simulink model "STEVE_Simulation"  (R2024b)
settings: Solver=ode4  StartTime=0.0  StopTime=60*6  FixedStep=0.05  RelTol=1e-3  EnableMultiTasking=on
values from neighbouring files (symbols this model uses):
  F = scatteredInterpolant(obj.MachData, obj.AlphaData, obj.CLData, obj.InterpMethod, 'none')    [LookupInitializer.m]
  rocket_length = max(STeVe_Contour.X) - min(STeVe_Contour.X)    [initialize_parameters.m]
  timeStep = 0.005    [initialize_parameters.m]
undefined symbols (not defined in the file or in its folder): Actuators, AeroData, Earth, Light, MIL, PrelookupData, Ref_Area, WGS84
libraries: aerolibwind2 x3, aerolibtransform2 x3, aerolibasang x3, simulink x1, aerolibatmos2 x1, simulink_extras x1, slpidlib x1, aerolibconvert2 x1, aerolibactuator x1
settings Model: ExtModeTrigDuration=2  Creator=jonno  LastModifiedBy=jonno
settings SolverCC: AutoInsertRateTranBlk=on
settings RTWCC: BuildConfiguration=Faster Runs

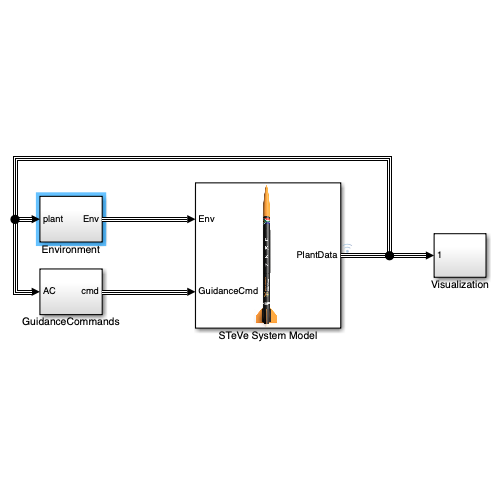
[thumbnail: Simulink's stored preview of the top-level diagram]
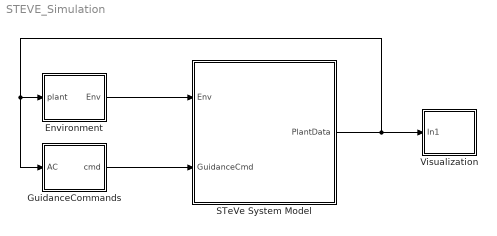
== system STEVE_Simulation ==
  Environment : Subsystem
  GuidanceCommands : Subsystem
  STeVe System Model : Subsystem
      mask Display: image('steve.png', [65 - (50 * (187 / 1041)), 0, 140 * (187 / 1041), 140])
  Visualization : Subsystem
  wires:
  GuidanceCommands/1(cmd) -> STeVe System Model/2(GuidanceCmd)
  Environment/1(Env) -> STeVe System Model/1(Env)
  STeVe System Model/1(PlantData) -> GuidanceCommands/1(AC), Environment/1(plant), Visualization/1(In1)

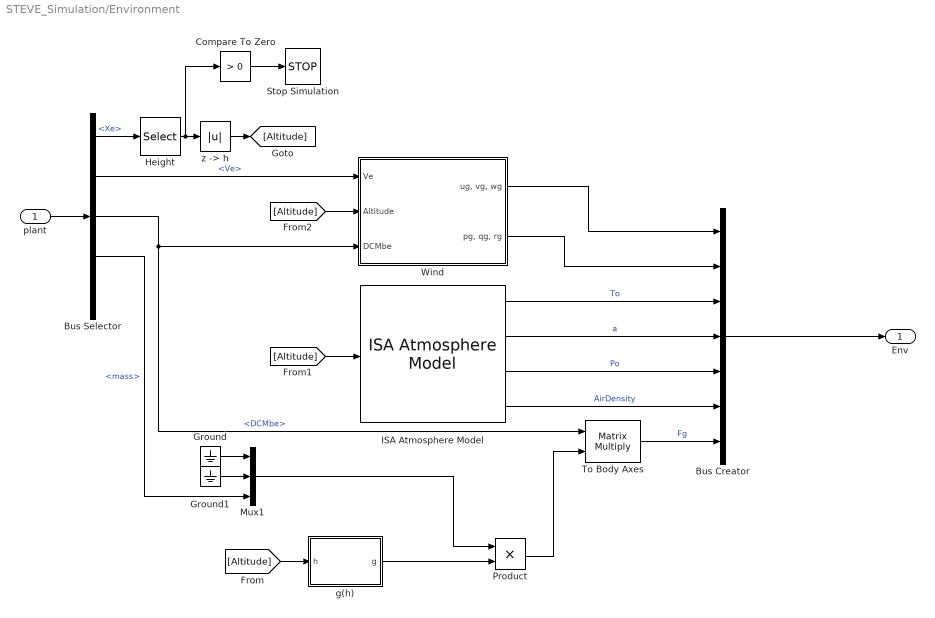
== system STEVE_Simulation/Environment ==
  plant : Inport
  Bus Creator : BusCreator  Inputs=7
  Bus Selector : BusSelector  OutputSignals=Xe,Ve,DCMbe,mass,lat
  Compare To Zero : simulink/Logic and Bit Operations/Compare To Zero  relop=>  OutDataTypeStr=boolean
  Ground : Ground
  Ground1 : Ground
  Height : Selector  IndexMode=Zero-based  InputPortWidth=3  IndexOptions=Index vector (dialog)  Indices=2  OutputSizes=1
  ISA Atmosphere Model : aerolibatmos2/ISA Atmosphere Model  useExtended=on  action=None  custom=off  viscosityOut=off  g=9.80665  gamma=1.4  R=287.0531  L=0.0065  h_trop=11000  h_strat=20000  rho0=1.225  P0=101325  T0=288.15  h0=0  S=110.4  Tref=273.15  muref=1.716e-5
  Mux1 : Mux  Inputs=3
  Product : Product
  Stop Simulation : Stop
  To Body Axes : Product  Multiplication=Matrix(*)
  Wind : Subsystem
  g(h) : MATLAB Function  TreatAsAtomicUnit=on
  "z -> h" : Abs  SaturateOnIntegerOverflow=off
  Env : Outport
  wires:
  plant/1 -> Bus Selector/1
  Bus Creator/1 -> Env/1
  Compare To Zero/1 -> Stop Simulation/1
  Bus Selector/1 -> Height/1  "<Xe>"
  Height/1 -> Compare To Zero/1, "z -> h"/1
  "z -> h"/1 -> [Altitude]
  Bus Selector/4 -> Mux1/3  "<mass>"
  Ground/1 -> Mux1/1
  Ground1/1 -> Mux1/2
  Bus Selector/3 -> Wind/3(DCMbe), To Body Axes/1  "<DCMbe>"
  [Altitude] -> ISA Atmosphere Model/1
  To Body Axes/1 -> Bus Creator/7  "Fg"
  ISA Atmosphere Model/4 -> Bus Creator/6  "AirDensity"
  ISA Atmosphere Model/3 -> Bus Creator/5  "Po"
  ISA Atmosphere Model/2 -> Bus Creator/4  "a"
  ISA Atmosphere Model/1 -> Bus Creator/3  "To"
  Bus Selector/2 -> Wind/1(Ve)  "<Ve>"
  [Altitude] -> Wind/2(Altitude)
  Wind/2("pg, qg, rg") -> Bus Creator/2
  Wind/1("ug, vg, wg") -> Bus Creator/1
  Mux1/1 -> Product/1
  Product/1 -> To Body Axes/2
  [Altitude] -> g(h)/1(h)
  g(h)/1(g) -> Product/2

== system STEVE_Simulation/GuidanceCommands ==
  AC : Inport
  Bus Creator : BusCreator  Inputs=2
  Degrees to Radians : simulink_extras/Transformations/Degrees to Radians
  Rate Limiter : RateLimiter  SampleTimeMode=inherited
  Terminator : Terminator
  ThetaCmd : Step  Before=90  After=90  SampleTime=0
  ThrottleCmd %1 : Step  Time=Actuators.Engine.BurnTime  Before=1  After=0  SampleTime=0
  cmd : Outport
  wires:
  AC/1 -> Terminator/1
  ThrottleCmd %1/1 -> Rate Limiter/1
  Bus Creator/1 -> cmd/1
  ThetaCmd/1 -> Degrees to Radians/1  "ThetaCmd"
  Degrees to Radians/1 -> Bus Creator/2  "ThetaCmd"
  Rate Limiter/1 -> Bus Creator/1  "ThrottleCmd"

== system STEVE_Simulation/STeVe System Model ==
  Env : Inport
  GuidanceCmd : Inport  Port=2
  Avionics : Subsystem
  Env1 : InportShadow
  Flight Sensors : Subsystem
  Vehicle : Subsystem
  PlantData : Outport
  wires:
  Env/1 -> Vehicle/1(Env)
  Vehicle/1(PlantData) -> Flight Sensors/2(Plant), Avionics/2(PlantData), PlantData/1  "Plant"
  Avionics/1(ActCmd) -> Vehicle/2(ActCmd)
  GuidanceCmd/1 -> Avionics/1(GuidanceCommandBus)
  Env1/1 -> Flight Sensors/1(Env)
  Flight Sensors/1(Sensors) -> Avionics/3(Sensors)

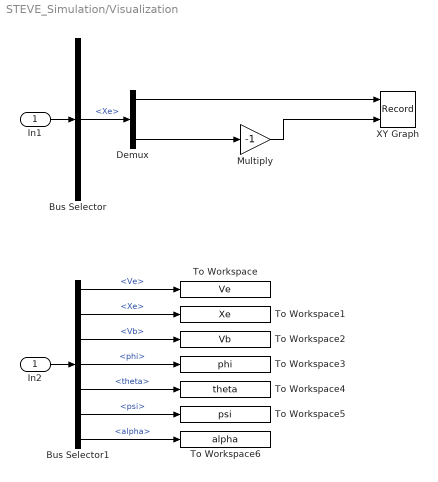
== system STEVE_Simulation/Visualization ==
  In1 : Inport
  Bus Selector : BusSelector  OutputSignals=Xe
  Bus Selector1 : BusSelector  OutputSignals=Ve,Xe,Vb,body angles.phi,body angles.theta,body angles.psi,alpha
  Demux : Demux  Outputs=3
  In2 : InportShadow
  Multiply : Gain  Gain=-1
  To Workspace : ToWorkspace  VariableName=Ve  SaveFormat=Timeseries  SampleTime=-1
  To Workspace1 : ToWorkspace  VariableName=Xe  SaveFormat=Timeseries  SampleTime=-1
  To Workspace2 : ToWorkspace  VariableName=Vb  SaveFormat=Timeseries  SampleTime=-1
  To Workspace3 : ToWorkspace  VariableName=phi  SaveFormat=Timeseries  SampleTime=-1
  To Workspace4 : ToWorkspace  VariableName=theta  SaveFormat=Timeseries  SampleTime=-1
  To Workspace5 : ToWorkspace  VariableName=psi  SaveFormat=Timeseries  SampleTime=-1
  To Workspace6 : ToWorkspace  VariableName=alpha  SaveFormat=Timeseries  SampleTime=-1
  XY Graph : Record  FileSettingsInternal="{\"entries\":[{\"content\":{\"excelSettings\":{\"content\":{},\"type\":\"Streamout.ExcelSettings\"}},\"type\":\"Streamout.FileSettingStorage\",\"uuid\":\"\"}],\"packageUris\":[\"http:\\/\\/schema.mathworks.com\\/mf0\\/streamout_blocks\\/R2020a\"],\"version\":\"1.0\"}"  Layout=[1 1]  SignalsInternal="{\"entries\":[{\"content\":{\"signals\":[{\"content\":{\"blockPath\":[],\"dimensions\":[1],\"domain\":\"\",\"lineColor\":\"#a2142f\",\"plots\":[ 1 ],\"port\":1,\"sid\":[\"\"],\"signalID\":1,\"signalName\":\"Demux:1\"},\"type\":\"RecordBlkView.Signal\",\"uuid\":\"\"},{\"content\":{\"blockPath\":[],\"dimensions\":[1],\"domain\":\"\",\"lineColor\":\"#139fff\",\"plots\":[ 1 ],\"port\":2,\"sid\":[\"\"],\"signalID\":2,\"signalName\":\"Multiply\"},\"type\":\"RecordBlkView.Signal\",\"uuid\":\"\"}]},\"type\":\"RecordBlkView.InputSignals\",\"uuid\":\"\"}],\"packageUris\":[\"http:\\/\\/schema.mathworks.com\\/mf0\\/streamout_blocks\\/R2020a\"],\"version\":\"1.0\"}"  VisualizationBindings="{\"xyplotplugin\":{\"info\":[{\"series\":[{\"bindingParametersList\":[{\"parameter\":\"X-Axis\",\"signalID\":1,\"signalName\":\"Demux:1\"},{\"parameter\":\"Y-Axis\",\"signalID\":2,\"signalName\":\"Multiply\"}],\"seriesID\":0}],\"subplotID\":1}]}}"  CompatibilityTag=XY
  wires:
  In1/1 -> Bus Selector/1
  Bus Selector/1 -> Demux/1  "<Xe>"
  Multiply/1 -> XY Graph/2
  Demux/3 -> Multiply/1
  Demux/1 -> XY Graph/1
  In2/1 -> Bus Selector1/1
  Bus Selector1/1 -> To Workspace/1  "<Ve>"
  Bus Selector1/2 -> To Workspace1/1  "<Xe>"
  Bus Selector1/3 -> To Workspace2/1  "<Vb>"
  Bus Selector1/4 -> To Workspace3/1  "<phi>"
  Bus Selector1/5 -> To Workspace4/1  "<theta>"
  Bus Selector1/6 -> To Workspace5/1  "<psi>"
  Bus Selector1/7 -> To Workspace6/1  "<alpha>"

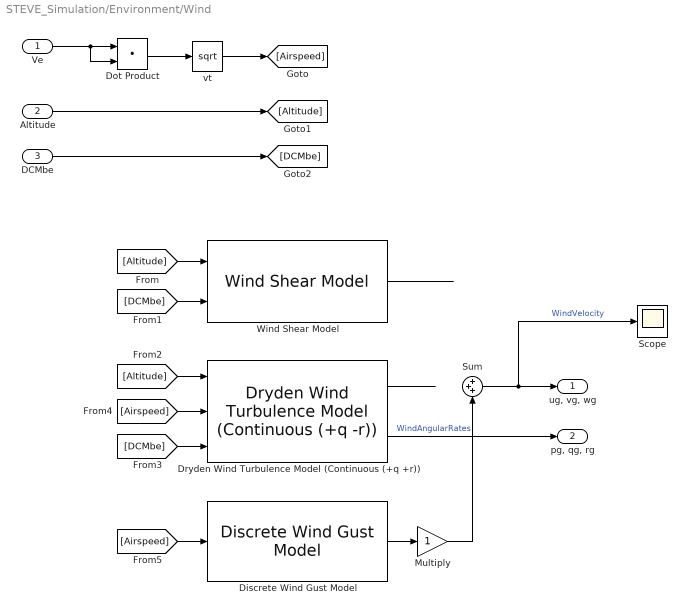
== system STEVE_Simulation/Environment/Wind ==
  Ve : Inport
  Altitude : Inport  Port=2
  DCMbe : Inport  Port=3
  Discrete Wind Gust Model : aerolibwind2/Discrete Wind Gust Model  units=Metric (MKS)  Gx=on  Gy=on  Gz=on  t_0=2  d_m=[120 100 80]  v_m=[3.5 4.0 3.0]
  Dot Product : DotProduct  OutDataTypeStr=Inherit: Inherit via internal rule
  Dryden Wind Turbulence Model (Continuous (+q +r)) : aerolibwind2/Dryden Wind Turbulence Model  (Continuous (+q -r))  units=Metric (MKS)  spec=MIL-F-8785C  model=Continuous Dryden (+q +r)  W20=15  Wdeg=0  TurbProb=10^-2 - Light  L_high=533.4  Wingspan=10  ts=0.1  Seed=[23341 23342 23343 23344]  T_on=off
      settings: LibrarySourceBlock=|
      | aerolibwind2/Dryden Wind Turbulence Model
      | (Continuous (+q +r))
  Multiply : Gain
  Scope : Scope
  Sum : Sum  Inputs=+++
  Wind Shear Model : aerolibwind2/Wind Shear Model  units=Metric (MKS)  phase=Category C - Terminal Flight Phase  W_20=1  Wdeg=0
  vt : Sqrt
  "ug, vg, wg" : Outport
  "pg, qg, rg" : Outport  Port=2
  wires:
  Ve/1 -> Dot Product/2, Dot Product/1
  Dot Product/1 -> vt/1
  vt/1 -> [Airspeed]
  DCMbe/1 -> [DCMbe]
  [Altitude] -> Wind Shear Model/1
  [DCMbe] -> Wind Shear Model/2
  [Altitude] -> Dryden Wind Turbulence Model (Continuous (+q +r))/1
  [DCMbe] -> Dryden Wind Turbulence Model (Continuous (+q +r))/3
  [Airspeed] -> Dryden Wind Turbulence Model (Continuous (+q +r))/2
  [Airspeed] -> Discrete Wind Gust Model/1
  Discrete Wind Gust Model/1 -> Multiply/1
  Wind Shear Model/1 -> ?
  Sum/1 -> Scope/1, "ug, vg, wg"/1  "WindVelocity"
  Dryden Wind Turbulence Model (Continuous (+q +r))/2 -> "pg, qg, rg"/1  "WindAngularRates"
  Altitude/1 -> [Altitude]
  Dryden Wind Turbulence Model (Continuous (+q +r))/1 -> ?
  Multiply/1 -> Sum/3

== system STEVE_Simulation/STeVe System Model/Avionics ==
  GuidanceCommandBus : Inport
  PlantData : Inport  Port=2
  Sensors : Inport  Port=3
  Bus Selector : BusSelector  OutputSignals=body angles.theta,w
  ControlSystem : Subsystem
  Scope : Scope
  ActCmd : Outport
  wires:
  PlantData/1 -> Bus Selector/1
  GuidanceCommandBus/1 -> ControlSystem/2(Guidance)
  ControlSystem/1(cmd) -> ActCmd/1
  Sensors/1 -> ?
  Bus Selector/1 -> ControlSystem/1(AvionicsBus), Scope/1  "<theta>"

== system STEVE_Simulation/STeVe System Model/Flight Sensors ==
  Env : Inport
  Plant : Inport  Port=2
  Sensors : Outport
  wires:
  Plant/1 -> ?

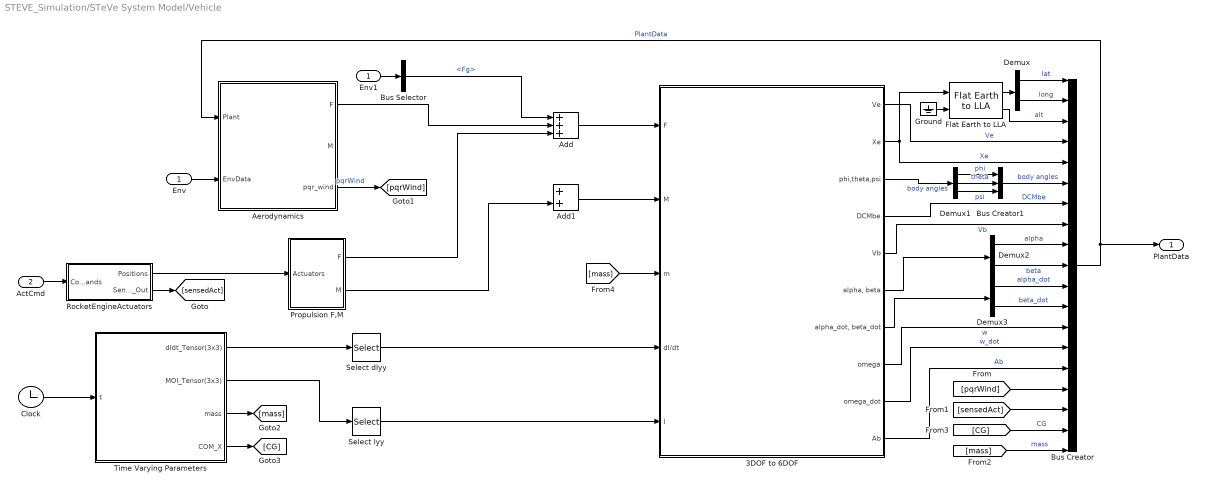
== system STEVE_Simulation/STeVe System Model/Vehicle ==
  Env : Inport
  ActCmd : Inport  Port=2
  3DOF to 6DOF : Subsystem
  Add : Sum  Inputs=+++
  Add1 : Sum
  Aerodynamics : Subsystem
  Bus Creator : BusCreator  Inputs=19
  Bus Creator1 : BusCreator  Inputs=3
  Bus Selector : BusSelector  OutputSignals=Fg
  Clock : Clock
  Demux : Demux  Outputs=2
  Demux1 : Demux  Outputs=3
  Demux2 : Demux  Outputs=2
  Demux3 : Demux  Outputs=2
  Env1 : InportShadow
  Flat Earth to LLA : aerolibtransform2/Flat Earth to LLA  units=Metric (MKS)  ptype=Earth (WGS84)  F=1/298.257223563  R=6378137  refPosPort=off  LL0=[0 10]  psi=0
  Ground : Ground
  Propulsion F,M : Subsystem
  RocketEngineActuators : Subsystem
  Select Iyy : Selector  NumberOfDimensions=2  InputPortWidth=3  IndexOptions=Index vector (dialog),Index vector (dialog)  Indices=[1],[1]  OutputSizes=1,1
  Select dIyy : Selector  NumberOfDimensions=2  InputPortWidth=3  IndexOptions=Index vector (dialog),Index vector (dialog)  Indices=[1],[1]  OutputSizes=1,1
  Time Varying Parameters : Subsystem
  PlantData : Outport
  wires:
  ActCmd/1 -> RocketEngineActuators/1(Commands)
  RocketEngineActuators/1(Positions) -> Propulsion F,M/1(Actuators)
  Bus Creator/1 -> Aerodynamics/1(Plant), PlantData/1  "PlantData"
  3DOF to 6DOF/2(Xe) -> Flat Earth to LLA/1, Bus Creator/5  "Xe"
  Demux/1 -> Bus Creator/1  "lat"
  Demux/2 -> Bus Creator/2  "long"
  Flat Earth to LLA/1 -> Demux/1
  Flat Earth to LLA/2 -> Bus Creator/3  "alt"
  Ground/1 -> Flat Earth to LLA/2
  3DOF to 6DOF/1(Ve) -> Bus Creator/4  "Ve"
  3DOF to 6DOF/3(phi,theta,psi) -> Demux1/1  "body angles"
  Demux1/1 -> Bus Creator1/1  "phi"
  Demux1/2 -> Bus Creator1/2  "theta"
  Demux1/3 -> Bus Creator1/3  "psi"
  Bus Creator1/1 -> Bus Creator/6  "body angles"
  3DOF to 6DOF/4(DCMbe) -> Bus Creator/7  "DCMbe"
  3DOF to 6DOF/5(Vb) -> Bus Creator/8  "Vb"
  3DOF to 6DOF/6("alpha, beta") -> Demux2/1
  Demux2/1 -> Bus Creator/9  "alpha"
  Demux2/2 -> Bus Creator/10  "beta"
  Demux3/2 -> Bus Creator/12  "beta_dot"
  Demux3/1 -> Bus Creator/11  "alpha_dot"
  3DOF to 6DOF/7("alpha_dot, beta_dot") -> Demux3/1
  3DOF to 6DOF/8(omega) -> Bus Creator/13  "w"
  3DOF to 6DOF/9(omega_dot) -> Bus Creator/14  "w_dot"
  3DOF to 6DOF/10(Ab) -> Bus Creator/15  "Ab"
  [pqrWind] -> Bus Creator/16
  [sensedAct] -> Bus Creator/17
  RocketEngineActuators/2(Sensed_Out) -> [sensedAct]
  Aerodynamics/3(pqr_wind) -> [pqrWind]  "pqrWind"
  Propulsion F,M/1(F) -> Add/3
  [CG] -> Bus Creator/18  "CG"
  [mass] -> Bus Creator/19  "mass"
  Env1/1 -> Bus Selector/1
  Bus Selector/1 -> Add/1  "<Fg>"
  Env/1 -> Aerodynamics/2(EnvData)
  Propulsion F,M/2(M) -> Add1/2
  Clock/1 -> Time Varying Parameters/1(t)
  Time Varying Parameters/1(dIdt_Tensor(3x3)) -> Select dIyy/1
  Select dIyy/1 -> 3DOF to 6DOF/4(dI/dt)
  Time Varying Parameters/2(MOI_Tensor(3x3)) -> Select Iyy/1
  Select Iyy/1 -> 3DOF to 6DOF/5(I)
  Time Varying Parameters/3(mass) -> [mass]
  Time Varying Parameters/4(COM_X) -> [CG]
  [mass] -> 3DOF to 6DOF/3(m)
  Add1/1 -> 3DOF to 6DOF/2(M)
  Add/1 -> 3DOF to 6DOF/1(F)
  Aerodynamics/1(F) -> Add/2

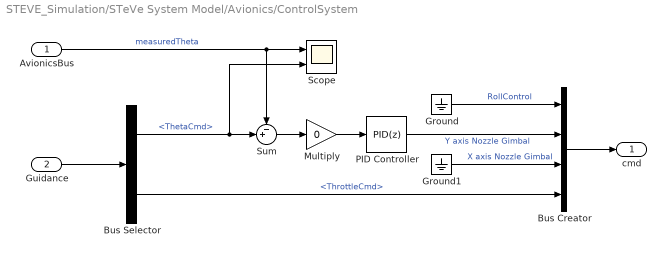
== system STEVE_Simulation/STeVe System Model/Avionics/ControlSystem ==
  AvionicsBus : Inport
  Guidance : Inport  Port=2
  Bus Creator : BusCreator  Inputs=4
  Bus Selector : BusSelector  OutputSignals=ThetaCmd,ThrottleCmd
  Ground : Ground
  Ground1 : Ground
  Multiply : Gain  Gain=0
  PID Controller : slpidlib/PID Controller  Controller=PID  Form=Parallel  TimeDomain=Discrete-time  UseExternalTs=off  SampleTime=-1  IntegratorMethod=Forward Euler  FilterMethod=Forward Euler  ControllerParametersSource=internal  P=3.36659028949205e-06  I=1.60713922295942e-07  UseKiTs=off  D=1.67830138926352e-05  UseExternalDerivativeSource=off  N=3.17121489439098  UseFilter=on  TunerSelectOption=Transfer Function Based (PID Tuner App)  InitialConditionSource=internal  InitialConditionForIntegrator=0  InitialConditionForFilter=0  DifferentiatorICPrevScaledInput=0  ExternalReset=none  TrackingMode=off  Kt=1  LimitOutput=off  SatLimitsSource=internal  UpperSaturationLimit=inf  LowerSaturationLimit=-inf  LinearizeAsGain=on  AntiWindupMode=none  Kb=1  LimitIntegrator=off  UpperIntegratorSaturationLimit=inf  LowerIntegratorSaturationLimit=-inf  POutMin=[]  POutMax=[]  IOutMin=[]  IOutMax=[]  DOutMin=[]  DOutMax=[]  NOutMin=[]  NOutMax=[]  SumOutMin=[]  SumOutMax=[]  SaturationOutMin=[]  SaturationOutMax=[]  PParamMin=[]  PParamMax=[]  IParamMin=[]  IParamMax=[]  DParamMin=[]  DParamMax=[]  NParamMin=[]  NParamMax=[]  KbParamMin=[]  KbParamMax=[]  KtParamMin=[]  KtParamMax=[]  KbOutMin=[]  KbOutMax=[]  KtOutMin=[]  KtOutMax=[]  IntegratorOutMin=[]  IntegratorOutMax=[]  FilterOutMin=[]  FilterOutMax=[]  SumI1OutMin=[]  SumI1OutMax=[]  SumI2OutMin=[]  SumI2OutMax=[]  SumI3OutMin=[]  SumI3OutMax=[]  SumI4OutMin=[]  SumI4OutMax=[]  SumDOutMin=[]  SumDOutMax=[]  DifferentiatorOutMin=[]  DifferentiatorOutMax=[]  FilterDiffOutCoefMin=[]  FilterDiffOutCoefMax=[]  ReciprocalOutMin=[]  ReciprocalOutMax=[]  SumDenOutMin=[]  SumDenOutMax=[]  SumNumOutMin=[]  SumNumOutMax=[]  DivideOutMin=[]  DivideOutMax=[]  UdiffTsProdOutMin=[]  UdiffTsProdOutMax=[]  NTsProdOutMin=[]  NTsProdOutMax=[]  UintegralTsProdOutMin=[]  UintegralTsProdOutMax=[]  UngainTsProdOutMin=[]  UngainTsProdOutMax=[]  ClampingZeroOutDataTypeStr=Inherit: Inherit via back propagation  ClampingZeroOutMin=[]  ClampingZeroOutMax=[]  FilterDenConstantOutDataTypeStr=Inherit: Inherit via back propagation  FilterDenConstantOutMin=[]  FilterDenConstantOutMax=[]  PCopyOutDataTypeStr=Inherit: Inherit via back propagation  PCopyOutMin=[]  PCopyOutMax=[]  NCopyOutDataTypeStr=Inherit: Inherit via back propagation  NCopyOutMin=[]  NCopyOutMax=[]  IntegratorContinuousStateAttributes=''  IntegratorStateMustResolveToSignalObject=off  IntegratorRTWStateStorageClass=Auto  FilterContinuousStateAttributes=''  FilterStateMustResolveToSignalObject=off  FilterRTWStateStorageClass=Auto  ParallelPVariant=InternalParameters  IdealPVariant=Disabled  IVariant=InternalParameters  DVariant=InternalParameters  IntegratorVariant=Discrete  SatVariant=Disabled  AWVariant=Passthrough  PCopyVariant=Disabled  TRVariant=Disabled  FdbkBlocksVariant=Forward  IdealPFdbkVariant=Disabled  SatFdbkVariant=Disabled  DerivativeFilterVariant=ForwardEulerFilter  NVariant=InternalParameters  NCopyVariant=Disabled  FilterICVariant=InternalICsFilter  IntegratorICVariant=InternalICs  ExternalResetVariant=Disabled  TRSumVariant=Passthrough  SumFdbkVariant=Disabled  SumVariant=Sum_PID  TsampFilterVariant=InternalTs  TsampNgainVariant=Passthrough  TsampIntegralVariant=Disabled_SignalSpec  ExternalSaturationOutDataTypeStr=Inherit: Same as second input  DerivativeSourceVariant=ErrorSignal  PreIntVariant=InternalPreInt
  Scope : Scope  NumInputPorts=2
  Sum : Sum  Inputs=-+|
  cmd : Outport
  wires:
  Bus Creator/1 -> cmd/1
  Ground/1 -> Bus Creator/1  "RollControl"
  PID Controller/1 -> Bus Creator/2  "Y axis Nozzle Gimbal"
  Ground1/1 -> Bus Creator/3  "X axis Nozzle Gimbal"
  Guidance/1 -> Bus Selector/1
  Bus Selector/2 -> Bus Creator/4  "<ThrottleCmd>"
  Bus Selector/1 -> Scope/2, Sum/2  "<ThetaCmd>"
  Sum/1 -> Multiply/1
  Multiply/1 -> PID Controller/1
  AvionicsBus/1 -> Scope/1, Sum/1  "measuredTheta"

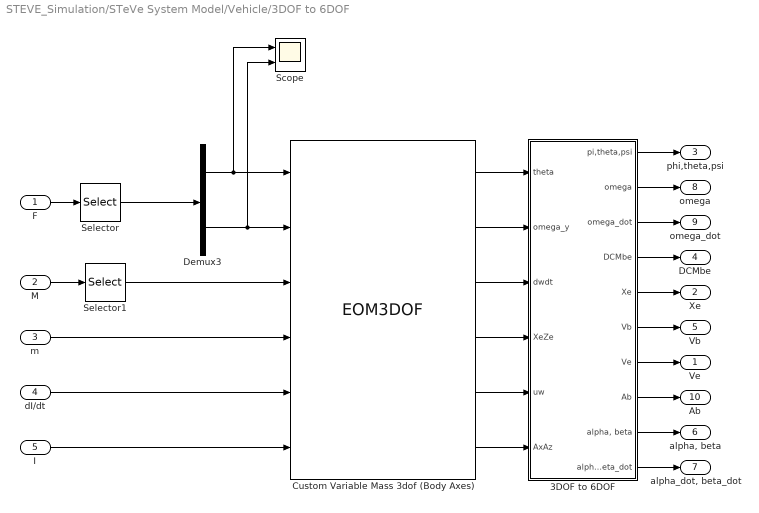
== system STEVE_Simulation/STeVe System Model/Vehicle/3DOF to 6DOF ==
  F : Inport
  M : Inport  Port=2
  m : Inport  Port=3
  dI/dt : Inport  Port=4
  I : Inport  Port=5
  3DOF to 6DOF : Subsystem
  Custom Variable Mass 3dof (Body Axes) : EOM3DOF  mtype=Custom Variable  v_ini=0  theta_ini=90*pi/180  g=0
  Demux3 : Demux  Outputs=2
  Scope : Scope  NumInputPorts=2
  Selector : Selector  InputPortWidth=3  IndexOptions=Index vector (dialog)  Indices=[1 3]  OutputSizes=1
  Selector1 : Selector  InputPortWidth=3  IndexOptions=Index vector (dialog)  Indices=[2]  OutputSizes=1
  Ve : Outport
  Xe : Outport  Port=2
  phi,theta,psi : Outport  Port=3
  DCMbe : Outport  Port=4
  Vb : Outport  Port=5
  "alpha, beta" : Outport  Port=6
  "alpha_dot, beta_dot" : Outport  Port=7
  omega : Outport  Port=8
  omega_dot : Outport  Port=9
  Ab : Outport  Port=10
  wires:
  F/1 -> Selector/1
  Demux3/2 -> Scope/2, Custom Variable Mass 3dof (Body Axes)/2
  Demux3/1 -> Scope/1, Custom Variable Mass 3dof (Body Axes)/1
  Selector/1 -> Demux3/1
  M/1 -> Selector1/1
  Selector1/1 -> Custom Variable Mass 3dof (Body Axes)/3
  Custom Variable Mass 3dof (Body Axes)/1 -> 3DOF to 6DOF/1(theta)
  Custom Variable Mass 3dof (Body Axes)/2 -> 3DOF to 6DOF/2(omega_y)
  Custom Variable Mass 3dof (Body Axes)/3 -> 3DOF to 6DOF/3(dwdt)
  Custom Variable Mass 3dof (Body Axes)/4 -> 3DOF to 6DOF/4(XeZe)
  Custom Variable Mass 3dof (Body Axes)/5 -> 3DOF to 6DOF/5(uw)
  Custom Variable Mass 3dof (Body Axes)/6 -> 3DOF to 6DOF/6(AxAz)
  3DOF to 6DOF/1(pi,theta,psi) -> phi,theta,psi/1
  3DOF to 6DOF/2(omega) -> omega/1
  3DOF to 6DOF/3(omega_dot) -> omega_dot/1
  3DOF to 6DOF/4(DCMbe) -> DCMbe/1
  3DOF to 6DOF/5(Xe) -> Xe/1
  3DOF to 6DOF/6(Vb) -> Vb/1
  3DOF to 6DOF/7(Ve) -> Ve/1
  3DOF to 6DOF/8(Ab) -> Ab/1
  3DOF to 6DOF/9("alpha, beta") -> "alpha, beta"/1
  3DOF to 6DOF/10("alpha_dot, beta_dot") -> "alpha_dot, beta_dot"/1
  I/1 -> Custom Variable Mass 3dof (Body Axes)/6
  dI/dt/1 -> Custom Variable Mass 3dof (Body Axes)/5
  m/1 -> Custom Variable Mass 3dof (Body Axes)/4

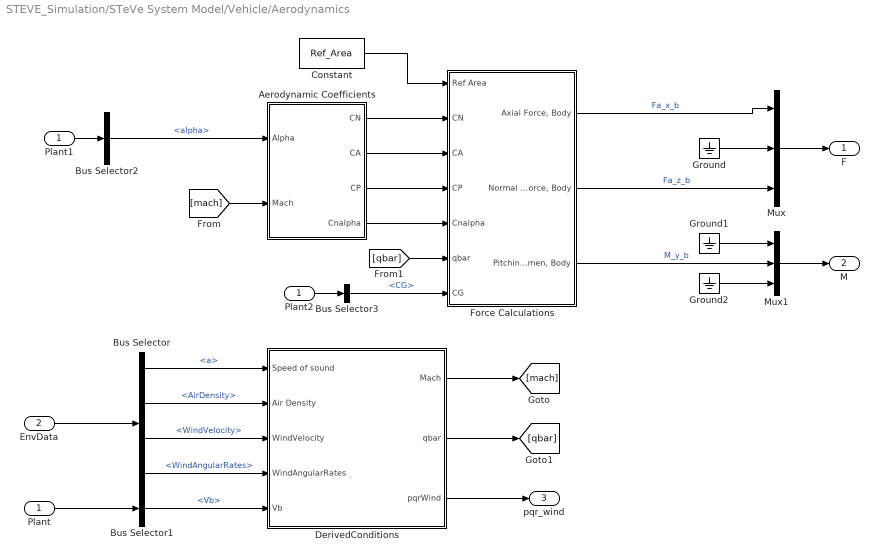
== system STEVE_Simulation/STeVe System Model/Vehicle/Aerodynamics ==
  Plant : Inport
  EnvData : Inport  Port=2
  Aerodynamic Coefficients : Subsystem
  Bus Selector : BusSelector  OutputSignals=a,AirDensity,WindVelocity,WindAngularRates
  Bus Selector1 : BusSelector  OutputSignals=Vb
  Bus Selector2 : BusSelector  OutputSignals=alpha
  Bus Selector3 : BusSelector  OutputSignals=CG
  Constant : Constant  Value=Ref_Area  VectorParams1D=off
  DerivedConditions : Subsystem
  Force Calculations : Subsystem
  Ground : Ground
  Ground1 : Ground
  Ground2 : Ground
  Mux : Mux  Inputs=3
  Mux1 : Mux  Inputs=3
  Plant1 : InportShadow
  Plant2 : InportShadow
  F : Outport
  M : Outport  Port=2
  pqr_wind : Outport  Port=3
  wires:
  Plant/1 -> Bus Selector1/1
  EnvData/1 -> Bus Selector/1
  Mux/1 -> F/1
  Ground2/1 -> Mux1/3
  Ground/1 -> Mux/2
  Force Calculations/2("Normal Force, Body") -> Mux/3  "Fa_z_b"
  Mux1/1 -> M/1
  Force Calculations/3("Pitching Momen, Body") -> Mux1/2  "M_y_b"
  Ground1/1 -> Mux1/1
  Force Calculations/1("Axial Force, Body") -> Mux/1  "Fa_x_b"
  Bus Selector1/1 -> DerivedConditions/5(Vb)  "<Vb>"
  Bus Selector/4 -> DerivedConditions/4(WindAngularRates)  "<WindAngularRates>"
  Bus Selector/3 -> DerivedConditions/3(WindVelocity)  "<WindVelocity>"
  Bus Selector/2 -> DerivedConditions/2(Air Density)  "<AirDensity>"
  Bus Selector/1 -> DerivedConditions/1(Speed of sound)  "<a>"
  DerivedConditions/1(Mach) -> [mach]
  DerivedConditions/2(qbar) -> [qbar]
  DerivedConditions/3(pqrWind) -> pqr_wind/1
  Plant1/1 -> Bus Selector2/1
  Bus Selector2/1 -> Aerodynamic Coefficients/1(Alpha)  "<alpha>"
  [mach] -> Aerodynamic Coefficients/2(Mach)
  Constant/1 -> Force Calculations/1(Ref Area)
  Aerodynamic Coefficients/1(CN) -> Force Calculations/2(CN)
  Aerodynamic Coefficients/2(CA) -> Force Calculations/3(CA)
  Aerodynamic Coefficients/3(CP) -> Force Calculations/4(CP)
  Aerodynamic Coefficients/4(Cnalpha) -> Force Calculations/5(Cnalpha)
  [qbar] -> Force Calculations/6(qbar)
  Plant2/1 -> Bus Selector3/1
  Bus Selector3/1 -> Force Calculations/7(CG)  "<CG>"

== system STEVE_Simulation/STeVe System Model/Vehicle/Propulsion F,M ==
  Actuators : Inport
  Bus Selector : BusSelector  OutputSignals=engineThrust,Y_nozzle_angle
  Ground : Ground
  Ground1 : Ground
  Ground2 : Ground
  MATLAB System : MATLABSystem  System=GimbalThrustModel  nozzleOffset=Actuators.Nozzle.MomentArm  SimulateUsing=Code generation
      mask Type: GimbalThrustModel
      mask Display:
      | disp('GimbalThrustModel');
      | port_label('input',1,'thrust');
      | port_label('input',2,'nozzle_angle');
      | port_label('output',1,'thrust_x');
      | port_label('output',2,'thrust_z');
      | port_label('output',3,'moment');
  Mux : Mux  Inputs=3
  Mux1 : Mux  Inputs=3
  Scope : Scope
  F : Outport
  M : Outport  Port=2
  wires:
  Actuators/1 -> Bus Selector/1
  Bus Selector/2 -> Scope/1, MATLAB System/2  "<Y_nozzle_angle>"
  Bus Selector/1 -> MATLAB System/1  "<engineThrust>"
  MATLAB System/3 -> Mux1/2  "M_y_b"
  MATLAB System/1 -> Mux/1  "Ft_x_b"
  MATLAB System/2 -> Mux/3  "Ft_z_b"
  Mux/1 -> F/1
  Ground/1 -> Mux/2
  Mux1/1 -> M/1
  Ground1/1 -> Mux1/1
  Ground2/1 -> Mux1/3

== system STEVE_Simulation/STeVe System Model/Vehicle/RocketEngineActuators ==
  Commands : Inport
  Bus Creator : BusCreator  Inputs=2
  Bus Selector : BusSelector  OutputSignals=Y axis Nozzle Gimbal,ThrottleCmd
  Multiply : Gain  Gain=Actuators.Engine.MaxThrust
  Multiply1 : Gain
  Nonlinear Second-Order Actuator : aerolibactuator/Nonlinear Second-Order Actuator  Commented=on  wn_fin=wn_act  z_fin=z_act  fin_max=maxdef_nozzle  fin_min=mindef_nozzle  fin_maxrate=rate_lim_nozzle  fin_act_0=0  fin_act_vel=0
  Positions : Outport
  Sensed_Out : Outport  Port=2
  wires:
  Commands/1 -> Bus Selector/1
  Bus Selector/1 -> Multiply1/1  "<Y axis Nozzle Gimbal>"
  Bus Creator/1 -> Sensed_Out/1, Positions/1  "Actuators"
  Bus Selector/2 -> Multiply/1  "<ThrottleCmd>"
  Multiply/1 -> Bus Creator/2  "engineThrust"
  Nonlinear Second-Order Actuator/1 -> ?  "Y_nozzle_angle"
  Multiply1/1 -> Bus Creator/1  "Y_nozzle_angle"

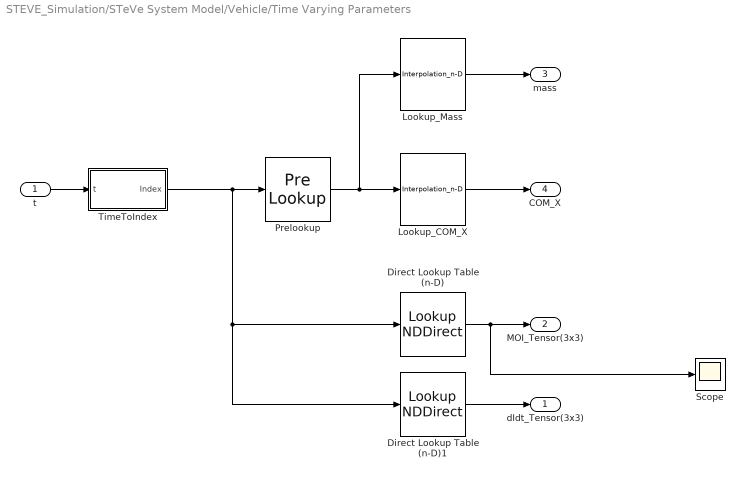
== system STEVE_Simulation/STeVe System Model/Vehicle/Time Varying Parameters ==
  t : Inport
  Direct Lookup Table (n-D) : LookupNDDirect  NumberOfTableDimensions=3  InputsSelectThisObjectFromTable=2-D Matrix  Table=PrelookupData.Tables.InertialTensor  DiagnosticForOutOfRangeInput=None  TableDataTypeStr=double
  Direct Lookup Table (n-D)1 : LookupNDDirect  NumberOfTableDimensions=3  InputsSelectThisObjectFromTable=2-D Matrix  Table=PrelookupData.Tables.dInertialTensor  DiagnosticForOutOfRangeInput=None  TableDataTypeStr=double
  Lookup_COM_X : Interpolation_n-D  NumberOfTableDimensions=1  Table=PrelookupData.Tables.COM_X  ExtrapMethod=Clip  DiagnosticForOutOfRangeInput=Warning  RequireIndexFractionAsBus=on  InternalRulePriority=Speed
      settings: InputPortMap=u0
  Lookup_Mass : Interpolation_n-D  NumberOfTableDimensions=1  Table=PrelookupData.Tables.Mass  ExtrapMethod=Clip  DiagnosticForOutOfRangeInput=Warning  RequireIndexFractionAsBus=on  OutDataTypeStr=double  InternalRulePriority=Speed  TableDataTypeStr=Inherit: Inherit from 'Table data'
      settings: InputPortMap=u0
  Prelookup : PreLookup  BreakpointsData=PrelookupData.Breakpoints.Index  OutputSelection=Index and fraction as bus  IndexSearchMethod=Evenly spaced points
  Scope : Scope
  TimeToIndex : Subsystem
  dIdt_Tensor(3x3) : Outport
  MOI_Tensor(3x3) : Outport  Port=2
  mass : Outport  Port=3
  COM_X : Outport  Port=4
  wires:
  Lookup_Mass/1 -> mass/1
  t/1 -> TimeToIndex/1(t)
  Lookup_COM_X/1 -> COM_X/1
  Direct Lookup Table (n-D)/1 -> Scope/1, MOI_Tensor(3x3)/1
  Direct Lookup Table (n-D)1/1 -> dIdt_Tensor(3x3)/1
  Prelookup/1 -> Lookup_Mass/1, Lookup_COM_X/1
  TimeToIndex/1(Index) -> Direct Lookup Table (n-D)/1, Direct Lookup Table (n-D)1/1, Prelookup/1

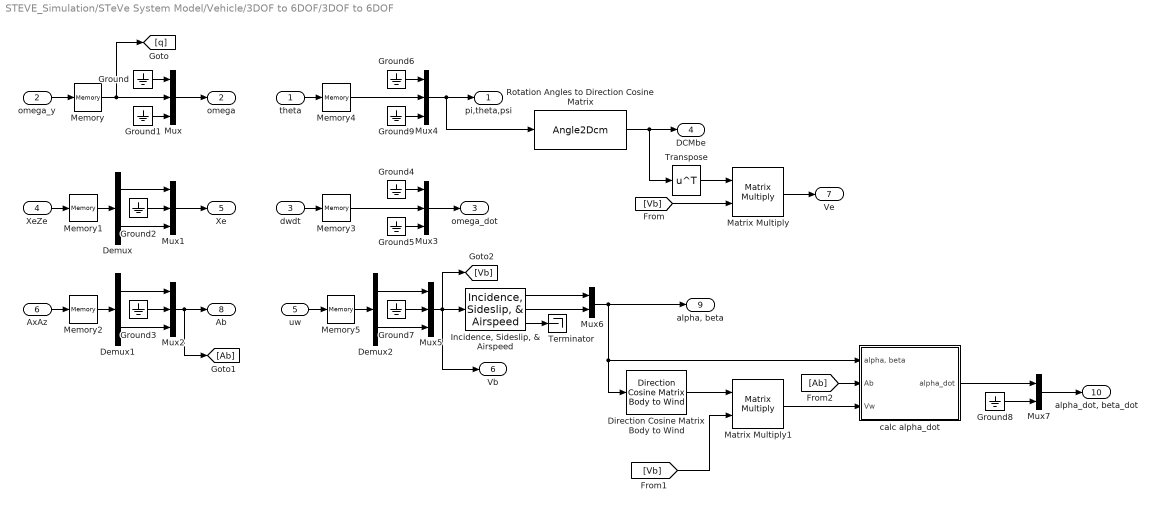
== system STEVE_Simulation/STeVe System Model/Vehicle/3DOF to 6DOF/3DOF to 6DOF ==
  theta : Inport
  omega_y : Inport  Port=2
  dwdt : Inport  Port=3
  XeZe : Inport  Port=4
  uw : Inport  Port=5
  AxAz : Inport  Port=6
  Demux : Demux  Outputs=2
  Demux1 : Demux  Outputs=2
  Demux2 : Demux  Outputs=2
  Direction Cosine Matrix Body to Wind : aerolibtransform2/Direction Cosine Matrix Body to Wind
  Ground{,1..9} (10 alike) : Ground
  "Incidence, Sideslip, & Airspeed" : aerolibasang/Incidence, Sideslip, & Airspeed
  Matrix Multiply : Product  Multiplication=Matrix(*)
  Matrix Multiply1 : Product  Multiplication=Matrix(*)
  Memory{,1..5} (6 alike) : Memory
  Mux{,1..5} (6 alike) : Mux  Inputs=3
  Mux6 : Mux  Inputs=2
  Mux7 : Mux  Inputs=2
  Rotation Angles to Direction Cosine Matrix : Angle2Dcm
      settings: AttributesFormatString=Rotation Order: %<rotationOrder>
      mask Display:
      | port_label('input',1,'[R_1,R_2,R_3]','texmode','on')
      | port_label('output',1,'DCM_{be}','texmode','on')
  Terminator : Terminator
  Transpose : Math  Operator=transpose
  calc alpha_dot : Subsystem
  pi,theta,psi : Outport
  omega : Outport  Port=2
  omega_dot : Outport  Port=3
  DCMbe : Outport  Port=4
  Xe : Outport  Port=5
  Vb : Outport  Port=6
  Ve : Outport  Port=7
  Ab : Outport  Port=8
  "alpha, beta" : Outport  Port=9
  "alpha_dot, beta_dot" : Outport  Port=10
  wires:
  omega_y/1 -> Memory/1
  Memory/1 -> [q], Mux/2
  Ground/1 -> Mux/1
  Ground1/1 -> Mux/3
  Demux/1 -> Mux1/1
  Ground2/1 -> Mux1/2
  Demux/2 -> Mux1/3
  Mux/1 -> omega/1
  XeZe/1 -> Memory1/1
  Memory1/1 -> Demux/1
  Mux1/1 -> Xe/1
  AxAz/1 -> Memory2/1
  Demux1/1 -> Mux2/1
  Demux1/2 -> Mux2/3
  Mux2/1 -> [Ab], Ab/1
  Memory2/1 -> Demux1/1
  Ground3/1 -> Mux2/2
  dwdt/1 -> Memory3/1
  Ground4/1 -> Mux3/1
  Ground5/1 -> Mux3/3
  Mux3/1 -> omega_dot/1
  Memory3/1 -> Mux3/2
  Ground9/1 -> Mux4/3
  Ground6/1 -> Mux4/1
  Mux4/1 -> Rotation Angles to Direction Cosine Matrix/1, pi,theta,psi/1
  theta/1 -> Memory4/1
  Memory4/1 -> Mux4/2
  Rotation Angles to Direction Cosine Matrix/1 -> Transpose/1, DCMbe/1
  Transpose/1 -> Matrix Multiply/1
  [Vb] -> Matrix Multiply/2
  Matrix Multiply/1 -> Ve/1
  uw/1 -> Memory5/1
  Demux2/2 -> Mux5/3
  Mux5/1 -> Vb/1, "Incidence, Sideslip, & Airspeed"/1, [Vb]
  Demux2/1 -> Mux5/1
  Ground7/1 -> Mux5/2
  Memory5/1 -> Demux2/1
  "Incidence, Sideslip, & Airspeed"/3 -> Terminator/1
  "Incidence, Sideslip, & Airspeed"/1 -> Mux6/1
  "Incidence, Sideslip, & Airspeed"/2 -> Mux6/2
  Mux6/1 -> calc alpha_dot/1("alpha, beta"), Direction Cosine Matrix Body to Wind/1, "alpha, beta"/1
  [Vb] -> Matrix Multiply1/2
  Direction Cosine Matrix Body to Wind/1 -> Matrix Multiply1/1
  Matrix Multiply1/1 -> calc alpha_dot/3(Vw)
  [Ab] -> calc alpha_dot/2(Ab)
  calc alpha_dot/1(alpha_dot) -> Mux7/1
  Ground8/1 -> Mux7/2
  Mux7/1 -> "alpha_dot, beta_dot"/1

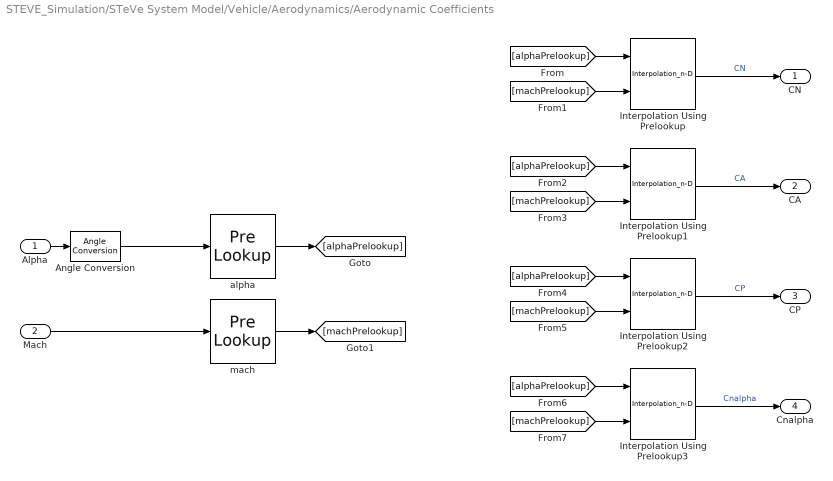
== system STEVE_Simulation/STeVe System Model/Vehicle/Aerodynamics/Aerodynamic Coefficients ==
  Alpha : Inport
  Mach : Inport  Port=2
  Angle Conversion : aerolibconvert2/Angle Conversion  IU=rad  OU=deg
  Interpolation Using Prelookup : Interpolation_n-D  Table=AeroData.Tables.CN  RequireIndexFractionAsBus=on  InternalRulePriority=Speed
      settings: InputPortMap=u0,u1
  Interpolation Using Prelookup1 : Interpolation_n-D  Table=AeroData.Tables.CAPower_On  RequireIndexFractionAsBus=on  InternalRulePriority=Speed
      settings: InputPortMap=u0,u1
  Interpolation Using Prelookup2 : Interpolation_n-D  Table=AeroData.Tables.CP  RequireIndexFractionAsBus=on  InternalRulePriority=Speed
      settings: InputPortMap=u0,u1
  Interpolation Using Prelookup3 : Interpolation_n-D  Table=AeroData.Tables.Cnalpha  RequireIndexFractionAsBus=on  InternalRulePriority=Speed
      settings: InputPortMap=u0,u1
  alpha : PreLookup  BreakpointsData=AeroData.Breakpoints.Alpha  OutputSelection=Index and fraction as bus  IndexSearchMethod=Evenly spaced points  ExtrapMethod=Linear
  mach : PreLookup  BreakpointsData=AeroData.Breakpoints.Mach  OutputSelection=Index and fraction as bus  IndexSearchMethod=Evenly spaced points  ExtrapMethod=Linear
  CN : Outport
  CA : Outport  Port=2
  CP : Outport  Port=3
  Cnalpha : Outport  Port=4
  wires:
  Interpolation Using Prelookup/1 -> CN/1  "CN"
  alpha/1 -> [alphaPrelookup]
  mach/1 -> [machPrelookup]
  [alphaPrelookup] -> Interpolation Using Prelookup/1
  [machPrelookup] -> Interpolation Using Prelookup/2
  Interpolation Using Prelookup1/1 -> CA/1  "CA"
  [machPrelookup] -> Interpolation Using Prelookup1/2
  [alphaPrelookup] -> Interpolation Using Prelookup1/1
  Interpolation Using Prelookup2/1 -> CP/1  "CP"
  [machPrelookup] -> Interpolation Using Prelookup2/2
  [alphaPrelookup] -> Interpolation Using Prelookup2/1
  Interpolation Using Prelookup3/1 -> Cnalpha/1  "Cnalpha"
  [machPrelookup] -> Interpolation Using Prelookup3/2
  [alphaPrelookup] -> Interpolation Using Prelookup3/1
  Alpha/1 -> Angle Conversion/1
  Angle Conversion/1 -> alpha/1
  Mach/1 -> mach/1

== system STEVE_Simulation/STeVe System Model/Vehicle/Aerodynamics/DerivedConditions ==
  Speed of sound : Inport
  Air Density : Inport  Port=2
  WindVelocity : Inport  Port=3
  WindAngularRates : Inport  Port=4
  Vb : Inport  Port=5
  Dynamic Pressure : aerolibasang/Dynamic Pressure
  Mach Number : aerolibasang/Mach Number
  Sum : Sum  Inputs=|++
  Mach : Outport
  qbar : Outport  Port=2
  pqrWind : Outport  Port=3
  wires:
  WindVelocity/1 -> Sum/2
  Vb/1 -> Sum/1
  Speed of sound/1 -> Mach Number/2
  Sum/1 -> Dynamic Pressure/1, Mach Number/1
  Mach Number/1 -> Mach/1  "Mach"
  Air Density/1 -> Dynamic Pressure/2
  Dynamic Pressure/1 -> qbar/1  "qbar"
  WindAngularRates/1 -> pqrWind/1

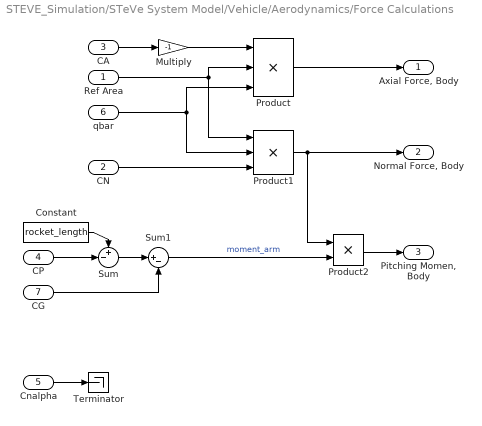
== system STEVE_Simulation/STeVe System Model/Vehicle/Aerodynamics/Force Calculations ==
  Ref Area : Inport
  CN : Inport  Port=2
  CA : Inport  Port=3
  CP : Inport  Port=4
  Cnalpha : Inport  Port=5
  qbar : Inport  Port=6
  CG : Inport  Port=7
  Constant : Constant  Value=rocket_length
  Multiply : Gain  Gain=-1
  Product : Product  Inputs=***
  Product1 : Product  Inputs=***
  Product2 : Product
  Sum : Sum  Inputs=+-|
  Sum1 : Sum  Inputs=|+-
  Terminator : Terminator
  "Axial Force, Body" : Outport
  "Normal Force, Body" : Outport  Port=2
  "Pitching Momen, Body" : Outport  Port=3
  wires:
  Product/1 -> "Axial Force, Body"/1
  CA/1 -> Multiply/1
  qbar/1 -> Product/3, Product1/2
  Ref Area/1 -> Product/2, Product1/1
  Multiply/1 -> Product/1
  Product1/1 -> Product2/1, "Normal Force, Body"/1
  CN/1 -> Product1/3
  Constant/1 -> Sum/1
  CP/1 -> Sum/2
  Sum/1 -> Sum1/1
  CG/1 -> Sum1/2
  Cnalpha/1 -> Terminator/1
  Sum1/1 -> Product2/2  "moment_arm"
  Product2/1 -> "Pitching Momen, Body"/1

== system STEVE_Simulation/STeVe System Model/Vehicle/Time Varying Parameters/TimeToIndex ==
  t : Inport
  Add Constant : Bias  Bias=1  SaturateOnIntegerOverflow=off
  Constant : Constant  Value=timeStep
  Product : Product  Inputs=*/
  Index : Outport
  wires:
  t/1 -> Product/1
  Constant/1 -> Product/2
  Product/1 -> Add Constant/1
  Add Constant/1 -> Index/1

== system STEVE_Simulation/STeVe System Model/Vehicle/3DOF to 6DOF/3DOF to 6DOF/calc alpha_dot ==
  "alpha, beta" : Inport
  Ab : Inport  Port=2
  Vw : Inport  Port=3
  "Add epsilon to avoid division by 0 " : Bias  Bias=1*10^-8  SaturateOnIntegerOverflow=off
  Direction Cosine Matrix Body to Wind : aerolibtransform2/Direction Cosine Matrix Body to Wind
  Matrix Multiply : Product  Multiplication=Matrix(*)
  Product : Product  Inputs=*/
  Selector : Selector  IndexMode=Zero-based  InputPortWidth=3  IndexOptions=Index vector (dialog)  Indices=2  OutputSizes=1
  Selector1 : Selector  IndexMode=Zero-based  InputPortWidth=3  IndexOptions=Index vector (dialog)  Indices=0  OutputSizes=1
  alpha_dot : Outport
  wires:
  "alpha, beta"/1 -> Direction Cosine Matrix Body to Wind/1
  Direction Cosine Matrix Body to Wind/1 -> Matrix Multiply/1
  Ab/1 -> Matrix Multiply/2
  Matrix Multiply/1 -> Selector/1
  Vw/1 -> Selector1/1
  Selector/1 -> Product/1
  Selector1/1 -> "Add epsilon to avoid division by 0 "/1
  Product/1 -> alpha_dot/1
  "Add epsilon to avoid division by 0 "/1 -> Product/2

== matlab function STEVE_Simulation/Environment/g(h) ==
  data: h input; g output
function g = fcn(h)
G = 6.67430*10^(-11);
M = 5.9722*10^(24);
R_e = 6.371*10^(6);

g = (G * M)/(R_e + h)^2;
